simulink model "lab2_EmulationSS_DiscreteTime_Nominal"  (R2020b)
settings: Solver=VariableStepAuto  StartTime=0.0  StopTime=10.0  RelTol=1e-3
undefined symbols (not defined in the file): Gamma0, H0, J0, K, Nu, Nx, Phi0, sens, stepAmplitude, Ts
settings Model: Creator=Musta  LastModifiedBy=Musta

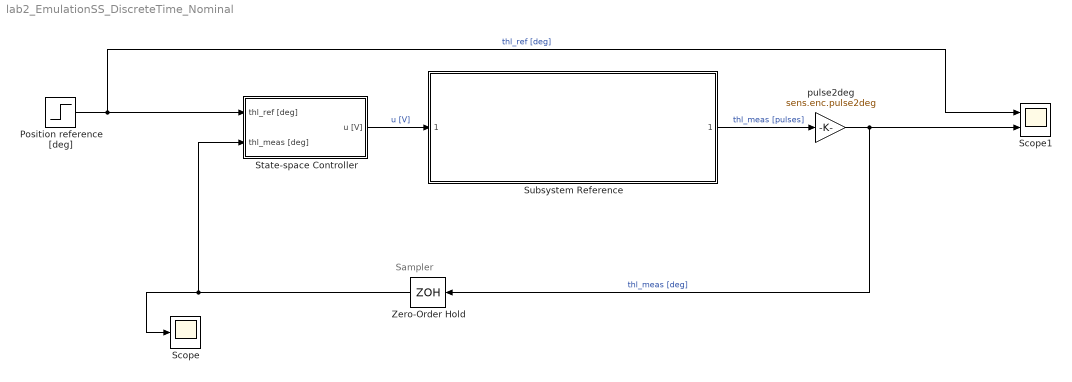
== system lab2_EmulationSS_DiscreteTime_Nominal ==
  note: Sampler
  Position reference [deg] : Step  Time=0  After=stepAmplitude  SampleTime=0
  Scope : Scope
  Scope1 : Scope  NumInputPorts=2
  State-space Controller : Subsystem
  Subsystem Reference : Subsystem  ReferencedSubsystem=plant_model
  Zero-Order Hold : ZeroOrderHold  SampleTime=Ts
  pulse2deg : Gain  Gain=sens.enc.pulse2deg
  wires:
  Position reference [deg]/1 -> Scope1/1, State-space Controller/1(thl_ref [deg])  "thl_ref [deg]"
  pulse2deg/1 -> Zero-Order Hold/1, Scope1/2  "thl_meas [deg]"
  Zero-Order Hold/1 -> Scope/1, State-space Controller/2(thl_meas [deg])
  State-space Controller/1(u [V]) -> Subsystem Reference/1  "u [V]"
  Subsystem Reference/1 -> pulse2deg/1  "thl_meas [pulses]"

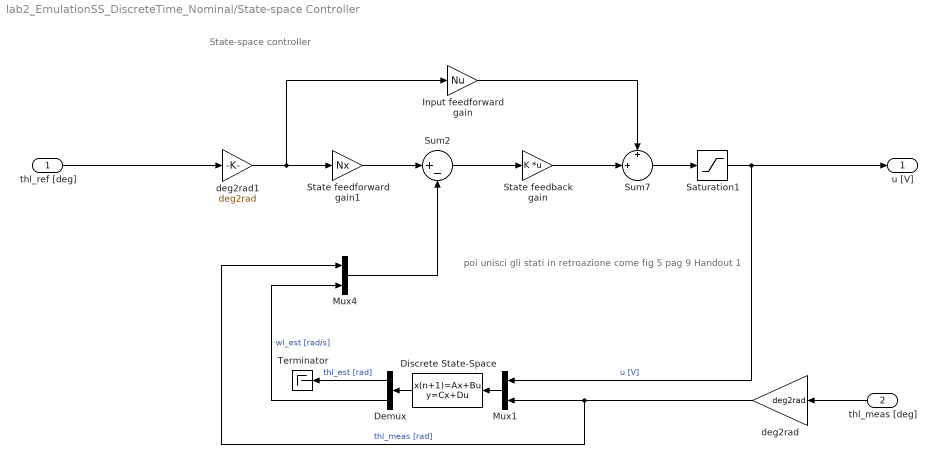
== system lab2_EmulationSS_DiscreteTime_Nominal/State-space Controller ==
  note: State-space controller
  note: poi unisci gli stati in retroazione come fig 5 pag 9 Handout 1
  thl_ref [deg] : Inport
  thl_meas [deg] : Inport  Port=2
  Demux : Demux  Outputs=2
  Discrete State-Space : DiscreteStateSpace  A=Phi0  B=Gamma0  C=H0  D=J0  SampleTime=Ts
  Input feedforward gain : Gain  Gain=Nu
  Mux1 : Mux  Inputs=2
  Mux4 : Mux  Inputs=2
  Saturation1 : Saturate  UpperLimit=12  LowerLimit=-12
  "State feedback gain " : Gain  Gain=K  Multiplication=Matrix(K*u)
  State feedforward gain1 : Gain  Gain=Nx
  Sum2 : Sum  Inputs=|+-
  Sum7 : Sum  Inputs=+|+||
  Terminator : Terminator
  deg2rad : Gain  Gain=deg2rad
  deg2rad1 : Gain  Gain=deg2rad
  u [V] : Outport
  wires:
  "State feedback gain "/1 -> Sum7/2
  thl_meas [deg]/1 -> deg2rad/1
  Sum7/1 -> Saturation1/1
  Input feedforward gain/1 -> Sum7/1
  deg2rad1/1 -> Input feedforward gain/1, State feedforward gain1/1
  Saturation1/1 -> u [V]/1, Mux1/1  "u [V]"
  Discrete State-Space/1 -> Demux/1
  Mux1/1 -> Discrete State-Space/1
  Sum2/1 -> "State feedback gain "/1
  State feedforward gain1/1 -> Sum2/1
  thl_ref [deg]/1 -> deg2rad1/1
  Demux/1 -> Terminator/1  "thl_est [rad]"
  deg2rad/1 -> Mux4/1, Mux1/2  "thl_meas [rad]"
  Demux/2 -> Mux4/2  "wl_est [rad/s]"
  Mux4/1 -> Sum2/2
